simulink model "L03"  (R2021a)
settings: Solver=FixedStepDiscrete  StartTime=0.0  StopTime=40.0  FixedStep=0.01  RelTol=1e-3
undefined symbols (not defined in the file): sigbuilder_block, Toff, Ton
settings Model: Creator=ncleju  LastModifiedBy=ncleju

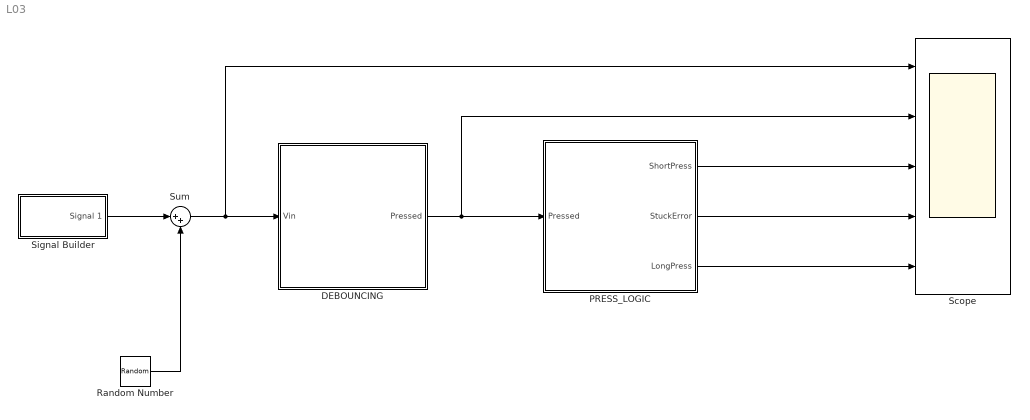
== system L03 ==
  DEBOUNCING : Stateflow chart  TreatAsAtomicUnit=on
  PRESS_LOGIC : Stateflow chart  TreatAsAtomicUnit=on
  Random Number : RandomNumber  Variance=0.001
  Scope : Scope  NumInputPorts=5
  Signal Builder : Subsystem  Tag=STV Subsys  LoadFcn=sigbuilder_block('load');  StartFcn=sigbuilder_block('start');  StopFcn=sigbuilder_block('stop');  ClipboardFcn=sigbuilder_block('clipboard');  mask(Sigbuilder block){tuvar=[0:10]}
      mask help: Simulink:masks:SigbuilderBlock_MD
      mask init:
      | if ~strcmp(get_param(bdroot(gcbh),'SimulationStatus'),'stopped') tuvar = sigbuilder_block('maskInit'); end
      settings: CopyFcn=sigbuilder_block('copy');  DeleteFcn=sigbuilder_block('delete');  ModelCloseFcn=sigbuilder_block('modelClose');  PreSaveFcn=sigbuilder_block('preSave');  PauseFcn=sigbuilder_block('pause');  ContinueFcn=sigbuilder_block('continue');  NameChangeFcn=sigbuilder_block('namechange');  OpenFcn=sigbuilder_block('open',[6 30 1428 681.75 ]);  CloseFcn=sigbuilder_block('close');
      mask Display: plot(0, 0, 100, 100,[2, 2, 32, 32, 2], [68, 8, 8, 68, 68],[32, 2], [38, 38], [32, 19, 2],[53, 60, 44], [32, 17, 17, 2],[16, 16, 31, 31]);txt = getActiveGroup(gcbh);text(2, 100, txt,'verticalAlignment', 'top');
  Sum : Sum  Inputs=|++
  wires:
  Sum/1 -> Scope/1, DEBOUNCING/1(Vin)
  Random Number/1 -> Sum/2
  Signal Builder/1(Signal 1) -> Sum/1
  DEBOUNCING/1(Pressed) -> Scope/2, PRESS_LOGIC/1(Pressed)
  PRESS_LOGIC/1(ShortPress) -> Scope/3
  PRESS_LOGIC/2(StuckError) -> Scope/4
  PRESS_LOGIC/3(LongPress) -> Scope/5

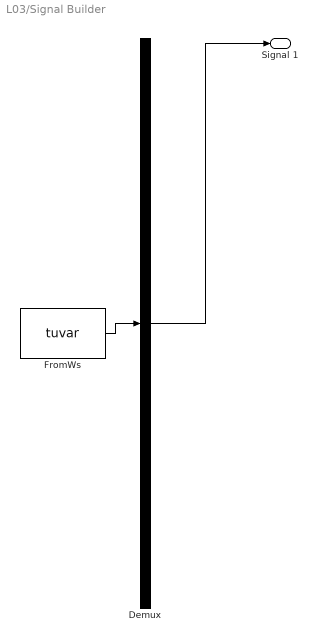
== system L03/Signal Builder ==
  Demux : Demux  Tag=STV Demux  Outputs=1
      settings: DisplayOption=none
  FromWs : FromWorkspace  Tag=STV FromWs  VariableName=tuvar
      SigBuilderData=|
      | common.afterFinalStr = 'Extrapolate'
      | common.sampleTime = 0
      | dataSet.timeRange = [0 40]
      | dataSet.name = 'Group 1'
      | sbobj.Groups.Name = 'Group 1'
      | sbobj.Groups.Signals.Name = 'Signal 1'
      | sbobj.Groups.Signals.XData = [0 0.17 0.18 0.7 0.76 0.76 0.84 0.86 0.9 0.98 0.98 1.98 2.08 3.98 4.1 5.98 6.08 6.12 6.24 6.28 6.34 10.7 11 12.35 12.55 40]
      | sbobj.Groups.Signals.YData = [4.99 5 0 0.02 4.94 0.02 0.02 4.98 0.02 0.02 5 5 0 0 5 5 0 4.97 0.01 4.79 0.02 0.01 5 5 0.01 -0.02]
      | sbobj.Groups.TimeRange = [0 40]
  Signal 1 : Outport  Tag=STV Outport
  wires:
  Demux/1 -> Signal 1/1
  FromWs/1 -> Demux/1

== stateflow chart L03/PRESS_LOGIC ==
  state IDLE
    en:
    ShortPress = false;
    LongPress = false;
    StuckError = false;
  state WAIT
  state SHORT
    en:
    ShortPress = true;
  state LONG_SUPERSTATE
    state LONG_OFF
      en:
      LongPress = false;
    state LONG_ON
      en:
      LongPress = true;
    (default) -> LONG_ON
    LONG_ON -> LONG_OFF : [after(Tout, msec)]
  state STUCK
    en:
    StuckError = true;
    LongPress = false;
  (default) -> IDLE
  (junction 17) -> IDLE
  (junction 16) -> (junction 17)
  IDLE -> WAIT : [Pressed==true]
  SHORT -> (junction 16) : [after(Tout, msec)]
  WAIT -> SHORT [order 1] : [Pressed == false]
  (junction 20) -> (junction 16)
  LONG_OFF -> (junction 20) : [Pressed == false]
  WAIT -> LONG_SUPERSTATE [order 2] : [after(3, sec)]
  (junction 26) -> (junction 20)
  LONG_SUPERSTATE -> STUCK : [after(22, sec)]
  STUCK -> (junction 26) : [Pressed == false]
  data: Pressed input; Tout parameter; ShortPress output; StuckError output; LongPress output

== stateflow chart L03/DEBOUNCING ==
  state OFF
    en:
    Pressed = false;
  state WAIT1
  state WAIT2
  state ON
    en:
    Pressed = true;
  (default) -> OFF
  OFF -> WAIT1 : [Vin < 0.5]
  WAIT1 -> OFF [order 1] : [Vin >= 0.5]
  WAIT2 -> OFF [order 2] : [after(Toff, msec)]
  WAIT1 -> ON [order 2] : [after(Ton, msec)]
  ON -> WAIT2 : [Vin > 4.5]
  WAIT2 -> ON [order 1] : [Vin <= 4.5]
  data: Ton parameter; Toff parameter; Vin input; Pressed output
